simulink model "HConstfolding_hier_export"  (Simulink 7.9)
settings: Solver=ode45  StartTime=0.0  StopTime=10.0  RelTol=1e-3
settings Model: Creator=boakes  LastModifiedBy=boakes

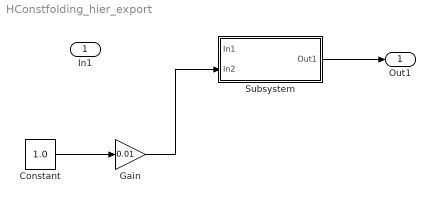
== system HConstfolding_hier_export ==
  In1 : Inport
  Constant : Constant  Value=1.0
  Gain : Gain  Gain=0.01
  Subsystem : Subsystem
  Out1 : Outport
  wires:
  Subsystem/1(Out1) -> Out1/1
  Constant/1 -> Gain/1
  Gain/1 -> Subsystem/2(In2)

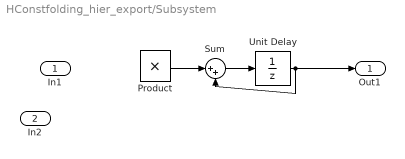
== system HConstfolding_hier_export/Subsystem ==
  In1 : Inport
  In2 : Inport  Port=2
  Product : Product  RndMeth=Zero
  Sum : Sum  Inputs=|++
  Unit Delay : UnitDelay  X0=0.0  SampleTime=-1.0
  Out1 : Outport
  wires:
  Product/1 -> Sum/1
  Sum/1 -> Unit Delay/1
  Unit Delay/1 -> Out1/1, Sum/2
